simulink model "modeltest"  (R2021a)
settings: Solver=VariableStepAuto  StartTime=0.0  StopTime=10.0  RelTol=1e-3
settings Model: Creator=Tyler  LastModifiedBy=Tyler

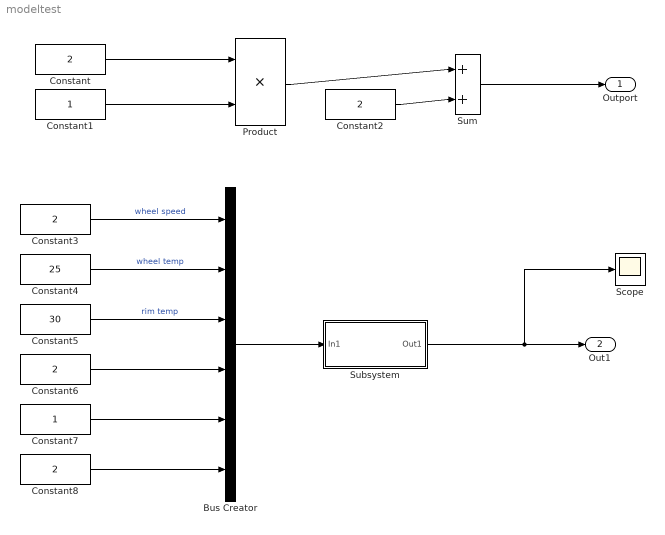
== system modeltest ==
  Bus Creator : BusCreator  Inputs=6
  Constant{,2..3,6,8} (5 alike) : Constant  Value=2
  Constant1 : Constant
  Constant4 : Constant  Value=25
  Constant5 : Constant  Value=30
  Constant7 : Constant
  Product : Product
  Scope : Scope
  Subsystem : Subsystem
  Sum : Sum  Inputs=|++
  Outport : Outport
  Out1 : Outport  Port=2
  wires:
  Constant/1 -> Product/1
  Constant1/1 -> Product/2
  Product/1 -> Sum/1
  Constant2/1 -> Sum/2
  Sum/1 -> Outport/1
  Constant4/1 -> Bus Creator/2  "wheel temp"
  Constant3/1 -> Bus Creator/1  "wheel speed"
  Constant5/1 -> Bus Creator/3  "rim temp"
  Constant6/1 -> Bus Creator/4
  Constant7/1 -> Bus Creator/5
  Constant8/1 -> Bus Creator/6
  Bus Creator/1 -> Subsystem/1(In1)
  Subsystem/1(Out1) -> Scope/1, Out1/1

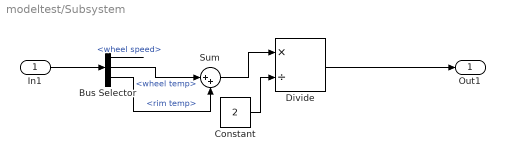
== system modeltest/Subsystem ==
  In1 : Inport
  Bus Selector : BusSelector  OutputSignals=wheel speed,wheel temp,rim temp
  Constant : Constant  Value=2
  Divide : Product  Inputs=*/
  Sum : Sum  Inputs=|++
  Out1 : Outport
  wires:
  In1/1 -> Bus Selector/1
  Bus Selector/1 -> ?  "<wheel speed>"
  Bus Selector/2 -> Sum/1  "<wheel temp>"
  Bus Selector/3 -> Sum/2  "<rim temp>"
  Sum/1 -> Divide/1
  Constant/1 -> Divide/2
  Divide/1 -> Out1/1
